simulink model "EST"  (R2024b)
settings: Solver=FixedStepAuto  StartTime=0.0  StopTime=stopt  FixedStep=deltat  MaxStep=0.05  RelTol=1e-3
InitFcn:
  | clear all;
  | close all;
  | clc;
  | 
  | % add the data and script directories
  | addpath('data','scripts');
  | 
  | % load the constants (units)
  | constants;
  | 
  | % load the simulation parameters
  | preprocessing;
StopFcn:
  | postprocessing;
values from neighbouring files (symbols this model uses):
  deltat = 15*unit("min")    [preprocessing.m]
undefined symbols (not defined in the file or in its folder): aElectricityDemand, aElectricToThermal, aExtraction, aInjection, alphaDemandTransport, aThermalToElectric, ccSurroundingsDemandTransport, ccSurroundingsStorage, ccSurroundingsSupplyTransport, dFluidDemandTransport, dFluidSupplyTransport, dStorageMaterial, eStorage, EStorageInitial, EStorageMax, EStorageMin, irPipeDemandTransport, irPipeSupplyTransport, l1PipeSupplyTransport, l2PipeSupplyTransport, lDemandTransport, lPipeDemandTransport, lStorage, rInjection, rplDemandTransport, rStorage, shcFluidDemandTransport, shcFluidSupplyTransport, shcStorageMaterial, tcInsDemandTransport, tcInsSupplyTransport, tcPipeDemandTransport, tcPipeSupplyTransport, tcStorage, tFluidSupplyTransport, tInsDemandTransport, tInsSupplyTransport, tMinStorage, tPipeDemandTransport, tPipeSupplyTransport, tStorage, tSurroundingsStorage, tSurroundingsSupplyTransport, vFluidDemandTransport, vFluidSupplyTransport
settings Model: Creator=joche  LastModifiedBy=nanda
settings DataIOCC: SaveFormat=Array  SaveOutput=off  ReturnWorkspaceOutputs=off
settings OptimizationCC: ReuseModelBlockBuffer=off
settings ModelReferenceCC: EnableRefExpFcnMdlSchedulingChecks=on
settings RTWCC: GPUComputeCapability=3.5

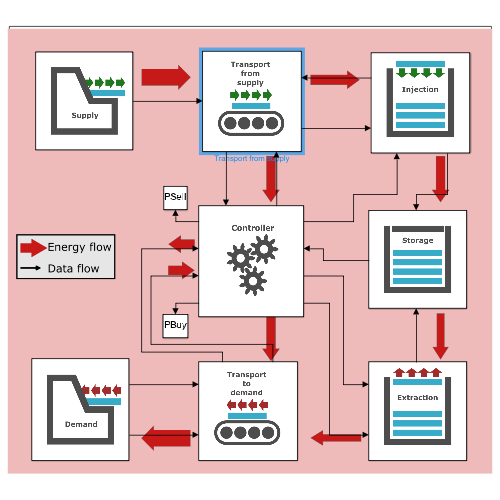
[thumbnail: Simulink's stored preview of the top-level diagram]
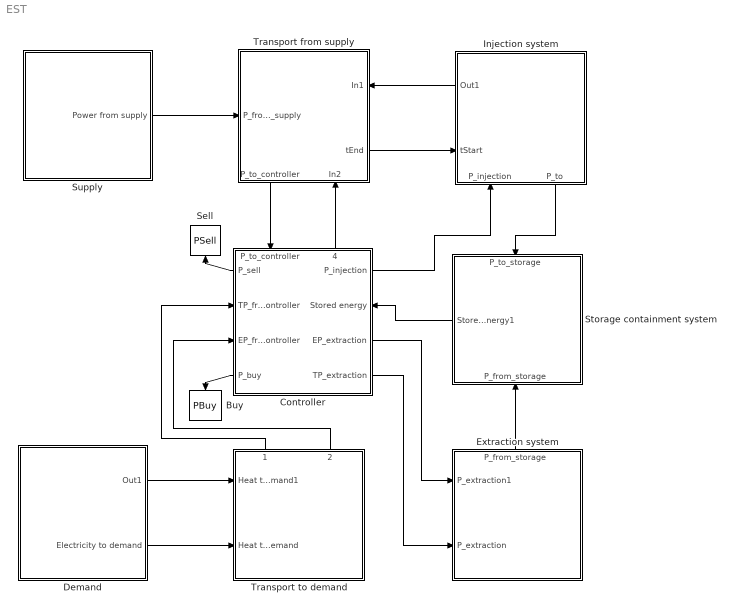
== system EST ==
  Buy : ToWorkspace  VariableName=PBuy  SampleTime=-1
  Controller : Subsystem
      settings: PortSchema="{\"entries\":[{\"content\":{\"sides\":[{\"content\":{\"connectorIds\":[\"Out5\",\"In1\",\"In2\",\"Out6\"]},\"type\":\"ConnectorPlacement.EquallySpacedRectSide\",\"uuid\":\"4656efb6-2d0d-4474-86b5-c32f145dee9d\"},{\"content\":{\"connectorIds\":[\"Out1\",\"In4\",\"Out2\",\"Out3\"],\"side\":\"RIGHT\"},\"type\":\"ConnectorPlacement.EquallySpacedRectSide\",\"uuid\":\"dff66aad-400a-439a-ac79-1f4b59d602b7\"},{\"content\":{\"connectorIds\":[\"In3\",\"Out4\"],\"side\":\"TOP\"},\"type\":\"ConnectorPlacement.EquallySpacedRectSide\",\"uuid\":\"e3dc4f2c-bed2-4e2c-ac62-d9db3cbbe72b\"}]},\"type\":\"ConnectorPlacement.EquallySpacedConnector\",\"uuid\":\"8904561c-f713-42e5-8c86-14541e4bd2e4\"}],\"packageUris\":[\"http://schema.mathworks.com/mf0/Connector/R2020b\"],\"version\":\"1.0\"}"
      mask Display: image('$imagefile'); % Use "Edit Image" on toolstrip to change.
  Demand : Subsystem
      mask Display: image('$imagefile'); % Use "Edit Image" on toolstrip to change.
  Extraction system : Subsystem
      settings: PortSchema="{\"entries\":[{\"content\":{\"sides\":[{\"content\":{},\"type\":\"ConnectorPlacement.EquallySpacedRectSide\",\"uuid\":\"05c5933d-55fc-4e06-853f-fc26d42905f9\"},{\"content\":{\"connectorIds\":[\"In1\",\"In2\"],\"side\":\"RIGHT\"},\"type\":\"ConnectorPlacement.EquallySpacedRectSide\",\"uuid\":\"327426c5-31d5-498b-a2bd-83e49353408c\"},{\"content\":{\"side\":\"TOP\"},\"type\":\"ConnectorPlacement.EquallySpacedRectSide\",\"uuid\":\"55306cf3-a3de-4385-a5ae-b8600ecdd5a2\"},{\"content\":{\"connectorIds\":[\"Out1\"],\"side\":\"BOTTOM\"},\"type\":\"ConnectorPlacement.EquallySpacedRectSide\",\"uuid\":\"08fcc9c3-40d3-4ac6-b914-dfeef6039ffb\"}]},\"type\":\"ConnectorPlacement.EquallySpacedConnector\",\"uuid\":\"cb35d5ba-e8c6-462c-b7b2-fe8356d4b0a1\"}],\"packageUris\":[\"http://schema.mathworks.com/mf0/Connector/R2020b\"],\"version\":\"1.0\"}"
      mask Display: image('$imagefile'); % Use "Edit Image" on toolstrip to change.
  Injection system : Subsystem
      settings: PortSchema="{\"entries\":[{\"content\":{\"sides\":[{\"content\":{},\"type\":\"ConnectorPlacement.EquallySpacedRectSide\",\"uuid\":\"05c5933d-55fc-4e06-853f-fc26d42905f9\"},{\"content\":{\"connectorIds\":[\"In2\",\"Out1\"],\"side\":\"RIGHT\"},\"type\":\"ConnectorPlacement.EquallySpacedRectSide\",\"uuid\":\"327426c5-31d5-498b-a2bd-83e49353408c\"},{\"content\":{\"connectorIds\":[\"Out2\",\"In1\"],\"side\":\"TOP\"},\"type\":\"ConnectorPlacement.EquallySpacedRectSide\",\"uuid\":\"55306cf3-a3de-4385-a5ae-b8600ecdd5a2\"},{\"content\":{\"side\":\"BOTTOM\"},\"type\":\"ConnectorPlacement.EquallySpacedRectSide\",\"uuid\":\"08fcc9c3-40d3-4ac6-b914-dfeef6039ffb\"}]},\"type\":\"ConnectorPlacement.EquallySpacedConnector\",\"uuid\":\"cb35d5ba-e8c6-462c-b7b2-fe8356d4b0a1\"}],\"packageUris\":[\"http://schema.mathworks.com/mf0/Connector/R2020b\"],\"version\":\"1.0\"}"
      mask Display: image('$imagefile'); % Use "Edit Image" on toolstrip to change.
  Sell : ToWorkspace  VariableName=PSell  SampleTime=-1
  Storage containment system : Subsystem
      settings: PortSchema="{\"entries\":[{\"content\":{\"sides\":[{\"content\":{\"connectorIds\":[\"Out1\"]},\"type\":\"ConnectorPlacement.EquallySpacedRectSide\",\"uuid\":\"0ba48424-33b9-4934-970f-64fe5d8b070e\"},{\"content\":{\"side\":\"RIGHT\"},\"type\":\"ConnectorPlacement.EquallySpacedRectSide\",\"uuid\":\"9cde340f-8f39-4499-9a12-5e1623737660\"},{\"content\":{\"connectorIds\":[\"In1\"],\"side\":\"TOP\"},\"type\":\"ConnectorPlacement.EquallySpacedRectSide\",\"uuid\":\"2af8db04-7fd0-4902-8637-8dc00edb4598\"},{\"content\":{\"connectorIds\":[\"In2\"],\"side\":\"BOTTOM\"},\"type\":\"ConnectorPlacement.EquallySpacedRectSide\",\"uuid\":\"e21ea806-d777-41a3-a53f-556fae66854b\"}]},\"type\":\"ConnectorPlacement.EquallySpacedConnector\",\"uuid\":\"4e2ddb36-4db3-4ab4-858b-ebb8ccefeb1f\"}],\"packageUris\":[\"http://schema.mathworks.com/mf0/Connector/R2020b\"],\"version\":\"1.0\"}"
      mask Display: image('$imagefile'); % Use "Edit Image" on toolstrip to change.
  Supply : Subsystem
      mask Display: image('$imagefile'); % Use "Edit Image" on toolstrip to change.
  Transport from supply : Subsystem
      settings: PortSchema="{\"entries\":[{\"content\":{\"sides\":[{\"content\":{\"connectorIds\":[\"In1\"]},\"type\":\"ConnectorPlacement.EquallySpacedRectSide\",\"uuid\":\"31329006-3d36-4d93-9c44-7503a515d397\"},{\"content\":{\"connectorIds\":[\"In3\",\"Out1\"],\"side\":\"RIGHT\"},\"type\":\"ConnectorPlacement.EquallySpacedRectSide\",\"uuid\":\"aba139c7-f9b6-4881-a56b-a4cbbedacd88\"},{\"content\":{\"side\":\"TOP\"},\"type\":\"ConnectorPlacement.EquallySpacedRectSide\",\"uuid\":\"e683eb73-7a35-4160-9c39-da83856a6278\"},{\"content\":{\"connectorIds\":[\"Out2\",\"In2\"],\"side\":\"BOTTOM\"},\"type\":\"ConnectorPlacement.EquallySpacedRectSide\",\"uuid\":\"1170dd18-447c-437f-9043-6812c2877331\"}]},\"type\":\"ConnectorPlacement.EquallySpacedConnector\",\"uuid\":\"804af608-1d70-444f-af69-e05f19bf98f3\"}],\"packageUris\":[\"http://schema.mathworks.com/mf0/Connector/R2020b\"],\"version\":\"1.0\"}"
      mask Display: image('$imagefile'); % Use "Edit Image" on toolstrip to change.
  Transport to demand : Subsystem
      settings: PortSchema="{\"entries\":[{\"content\":{\"sides\":[{\"content\":{\"connectorIds\":[\"In1\",\"In2\"]},\"type\":\"ConnectorPlacement.EquallySpacedRectSide\",\"uuid\":\"31329006-3d36-4d93-9c44-7503a515d397\"},{\"content\":{\"side\":\"RIGHT\"},\"type\":\"ConnectorPlacement.EquallySpacedRectSide\",\"uuid\":\"aba139c7-f9b6-4881-a56b-a4cbbedacd88\"},{\"content\":{\"connectorIds\":[\"Out1\",\"Out2\"],\"side\":\"TOP\"},\"type\":\"ConnectorPlacement.EquallySpacedRectSide\",\"uuid\":\"e683eb73-7a35-4160-9c39-da83856a6278\"},{\"content\":{\"side\":\"BOTTOM\"},\"type\":\"ConnectorPlacement.EquallySpacedRectSide\",\"uuid\":\"c378138f-7233-4483-870c-40a69b3495ee\"}]},\"type\":\"ConnectorPlacement.EquallySpacedConnector\",\"uuid\":\"804af608-1d70-444f-af69-e05f19bf98f3\"}],\"packageUris\":[\"http://schema.mathworks.com/mf0/Connector/R2020b\"],\"version\":\"1.0\"}"
      mask Display: image('$imagefile'); % Use "Edit Image" on toolstrip to change.
  wires:
  Supply/1(Power from supply) -> Transport from supply/1(P_from_supply)
  Transport from supply/2(P_to_controller) -> Controller/3(P_to_controller)
  Transport to demand/1(P_from_controler) -> Controller/1(TP_from_controller)
  Demand/1(Out1) -> Transport to demand/1(Heat to demand1)
  Controller/3(TP_extraction) -> Extraction system/1(P_extraction)
  Injection system/2(P_to) -> Storage containment system/1(P_to_storage)
  Extraction system/1(P_from_storage) -> Storage containment system/2(P_from_storage)
  Storage containment system/1(Stored energy1) -> Controller/4(Stored energy)
  Controller/1(P_injection) -> Injection system/1(P_injection)
  Controller/6(P_buy) -> Buy/1
  Transport from supply/1(tEnd) -> Injection system/2(tStart)
  Controller/5(P_sell) -> Sell/1
  Injection system/1(Out1) -> Transport from supply/3(In1)
  Demand/2(Electricity to demand) -> Transport to demand/2(Heat to demand)
  Transport to demand/2(P_from_controler1) -> Controller/2(EP_from_controller)
  Controller/2(EP_extraction) -> Extraction system/2(P_extraction1)
  Controller/4(TP_sold_from_pipes) -> Transport from supply/2(In2)

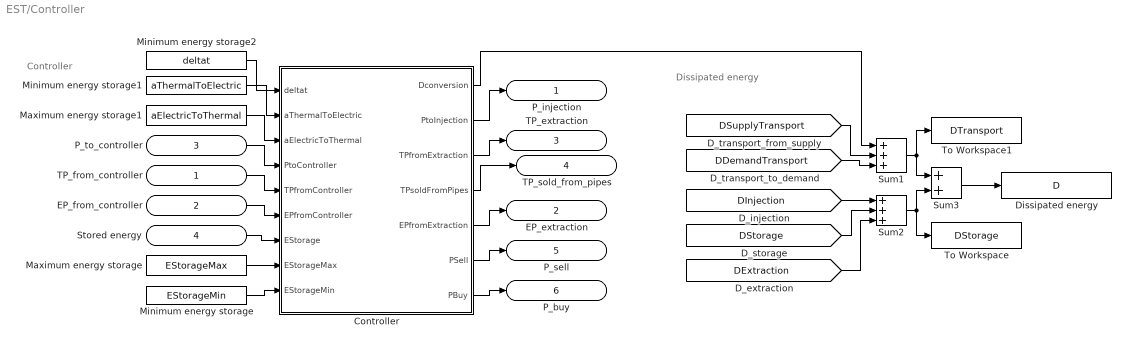
== system EST/Controller ==
  note: Dissipated energy
  note: Controller
  TP_from_controller : Inport
  EP_from_controller : Inport  Port=2
  P_to_controller : Inport  Port=3
  Stored energy : Inport  Port=4
  Controller : MATLAB Function  TreatAsAtomicUnit=on
  Dissipated energy : ToWorkspace  VariableName=D  SampleTime=-1
  Maximum energy storage : Constant  Value=EStorageMax
  Maximum energy storage1 : Constant  Value=aElectricToThermal
  Minimum energy storage : Constant  Value=EStorageMin
  Minimum energy storage1 : Constant  Value=aThermalToElectric
  Minimum energy storage2 : Constant  Value=deltat
  Sum1 : Sum  Inputs=+++
  Sum2 : Sum  Inputs=+++
  Sum3 : Sum
  To Workspace : ToWorkspace  VariableName=DStorage  SampleTime=-1
  To Workspace1 : ToWorkspace  VariableName=DTransport  SampleTime=-1
  P_injection : Outport
  EP_extraction : Outport  Port=2
  TP_extraction : Outport  Port=3
  TP_sold_from_pipes : Outport  Port=4
  P_sell : Outport  Port=5
  P_buy : Outport  Port=6
  wires:
  TP_from_controller/1 -> Controller/5(TPfromController)
  Controller/3(TPfromExtraction) -> TP_extraction/1
  Controller/6(PSell) -> P_sell/1
  Controller/7(PBuy) -> P_buy/1
  Minimum energy storage/1 -> Controller/9(EStorageMin)
  Maximum energy storage/1 -> Controller/8(EStorageMax)
  P_to_controller/1 -> Controller/4(PtoController)
  Controller/2(PtoInjection) -> P_injection/1
  Stored energy/1 -> Controller/7(EStorage)
  [DDemandTransport] -> Sum1/3
  [DSupplyTransport] -> Sum1/2
  [DInjection] -> Sum2/1
  [DStorage] -> Sum2/2
  [DExtraction] -> Sum2/3
  Sum2/1 -> To Workspace/1, Sum3/2
  Sum1/1 -> To Workspace1/1, Sum3/1
  Sum3/1 -> Dissipated energy/1
  EP_from_controller/1 -> Controller/6(EPfromController)
  Controller/5(EPfromExtraction) -> EP_extraction/1
  Maximum energy storage1/1 -> Controller/3(aElectricToThermal)
  Minimum energy storage1/1 -> Controller/2(aThermalToElectric)
  Controller/1(Dconversion) -> Sum1/1
  Minimum energy storage2/1 -> Controller/1(deltat)
  Controller/4(TPsoldFromPipes) -> TP_sold_from_pipes/1

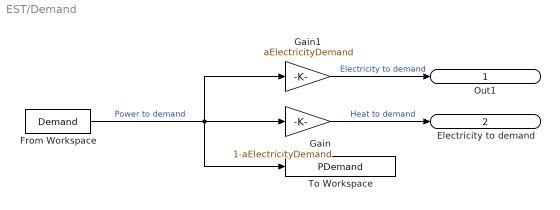
== system EST/Demand ==
  From Workspace : FromWorkspace  VariableName=Demand  OutputAfterFinalValue=Setting to zero
  Gain : Gain  Gain=1-aElectricityDemand
  Gain1 : Gain  Gain=aElectricityDemand
  To Workspace : ToWorkspace  VariableName=PDemand  SampleTime=-1
  Out1 : Outport
  Electricity to demand : Outport  Port=2
  wires:
  From Workspace/1 -> Gain/1, Gain1/1, To Workspace/1  "Power to demand"
  Gain/1 -> Electricity to demand/1  "Heat to demand"
  Gain1/1 -> Out1/1  "Electricity to demand"

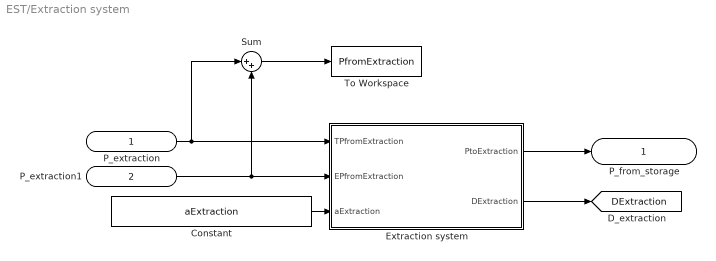
== system EST/Extraction system ==
  P_extraction : Inport
  P_extraction1 : Inport  Port=2
  Constant : Constant  Value=aExtraction
  Extraction system : MATLAB Function  TreatAsAtomicUnit=on
  Sum : Sum  Inputs=|++
  To Workspace : ToWorkspace  VariableName=PfromExtraction  SampleTime=-1
  P_from_storage : Outport
  tag scope: DExtraction=global
  wires:
  P_extraction/1 -> Sum/1, Extraction system/1(TPfromExtraction)
  Extraction system/1(PtoExtraction) -> P_from_storage/1
  Extraction system/2(DExtraction) -> [DExtraction]
  Constant/1 -> Extraction system/3(aExtraction)
  P_extraction1/1 -> Extraction system/2(EPfromExtraction), Sum/2
  Sum/1 -> To Workspace/1

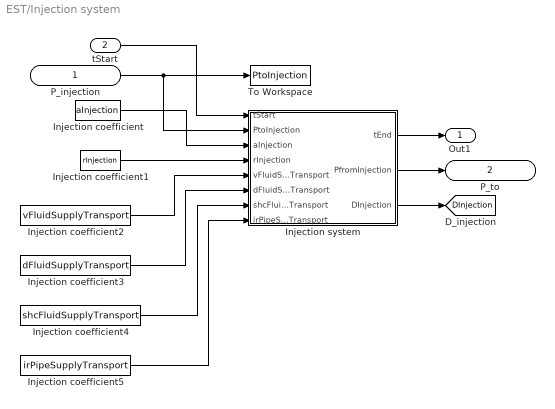
== system EST/Injection system ==
  P_injection : Inport
  tStart : Inport  Port=2
  Injection coefficient : Constant  Value=aInjection
  Injection coefficient1 : Constant  Value=rInjection
  Injection coefficient2 : Constant  Value=vFluidSupplyTransport
  Injection coefficient3 : Constant  Value=dFluidSupplyTransport
  Injection coefficient4 : Constant  Value=shcFluidSupplyTransport
  Injection coefficient5 : Constant  Value=irPipeSupplyTransport
  Injection system : MATLAB Function  TreatAsAtomicUnit=on
  To Workspace : ToWorkspace  VariableName=PtoInjection  SampleTime=-1
  Out1 : Outport
  P_to : Outport  Port=2
  tag scope: DInjection=global
  wires:
  Injection coefficient4/1 -> Injection system/7(shcFluidSupplyTransport)
  Injection coefficient1/1 -> Injection system/4(rInjection)
  tStart/1 -> Injection system/1(tStart)
  P_injection/1 -> To Workspace/1, Injection system/2(PtoInjection)
  Injection coefficient/1 -> Injection system/3(aInjection)
  Injection coefficient2/1 -> Injection system/5(vFluidSupplyTransport)
  Injection coefficient3/1 -> Injection system/6(dFluidSupplyTransport)
  Injection coefficient5/1 -> Injection system/8(irPipeSupplyTransport)
  Injection system/1(tEnd) -> Out1/1
  Injection system/2(PfromInjection) -> P_to/1
  Injection system/3(DInjection) -> [DInjection]

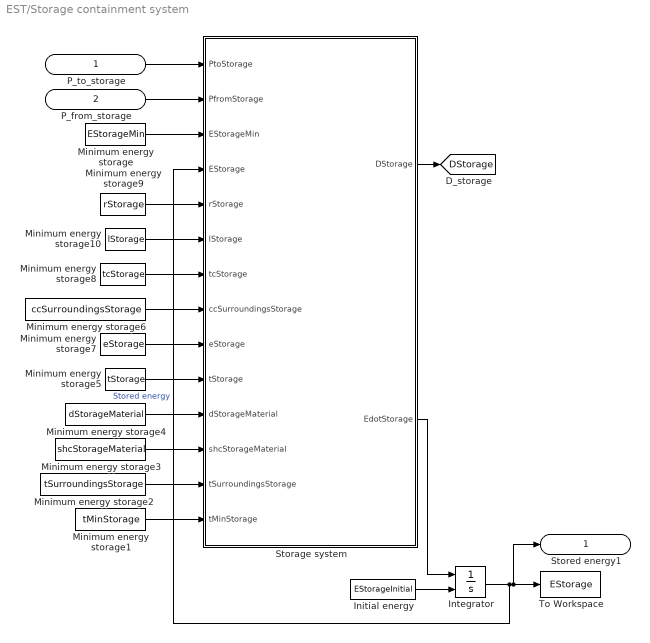
== system EST/Storage containment system ==
  P_to_storage : Inport
  P_from_storage : Inport  Port=2
  Initial energy : Constant  Value=EStorageInitial
  Integrator : Integrator  InitialConditionSource=external
  Minimum energy storage : Constant  Value=EStorageMin
  Minimum energy storage1 : Constant  Value=tMinStorage
  Minimum energy storage10 : Constant  Value=lStorage
  Minimum energy storage2 : Constant  Value=tSurroundingsStorage
  Minimum energy storage3 : Constant  Value=shcStorageMaterial
  Minimum energy storage4 : Constant  Value=dStorageMaterial
  Minimum energy storage5 : Constant  Value=tStorage
  Minimum energy storage6 : Constant  Value=ccSurroundingsStorage
  Minimum energy storage7 : Constant  Value=eStorage
  Minimum energy storage8 : Constant  Value=tcStorage
  Minimum energy storage9 : Constant  Value=rStorage
  Storage system : MATLAB Function  TreatAsAtomicUnit=on
  To Workspace : ToWorkspace  VariableName=EStorage  SampleTime=-1
  Stored energy1 : Outport
  tag scope: DStorage=global
  wires:
  P_from_storage/1 -> Storage system/2(PfromStorage)
  Initial energy/1 -> Integrator/2
  P_to_storage/1 -> Storage system/1(PtoStorage)
  Minimum energy storage3/1 -> Storage system/12(shcStorageMaterial)
  Minimum energy storage/1 -> Storage system/3(EStorageMin)
  Minimum energy storage7/1 -> Storage system/9(eStorage)
  Minimum energy storage2/1 -> Storage system/13(tSurroundingsStorage)
  Minimum energy storage6/1 -> Storage system/8(ccSurroundingsStorage)
  Minimum energy storage5/1 -> Storage system/10(tStorage)
  Minimum energy storage10/1 -> Storage system/6(lStorage)
  Minimum energy storage8/1 -> Storage system/7(tcStorage)
  Minimum energy storage9/1 -> Storage system/5(rStorage)
  Minimum energy storage1/1 -> Storage system/14(tMinStorage)
  Minimum energy storage4/1 -> Storage system/11(dStorageMaterial)
  Storage system/1(DStorage) -> [DStorage]
  Storage system/2(EdotStorage) -> Integrator/1
  Integrator/1 -> To Workspace/1, Stored energy1/1, Storage system/4(EStorage)  "Stored energy"

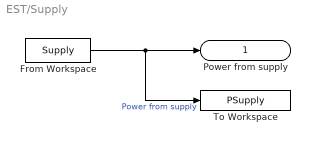
== system EST/Supply ==
  From Workspace : FromWorkspace  VariableName=Supply
  To Workspace : ToWorkspace  VariableName=PSupply  SampleTime=-1
  Power from supply : Outport
  wires:
  From Workspace/1 -> To Workspace/1, Power from supply/1  "Power from supply"

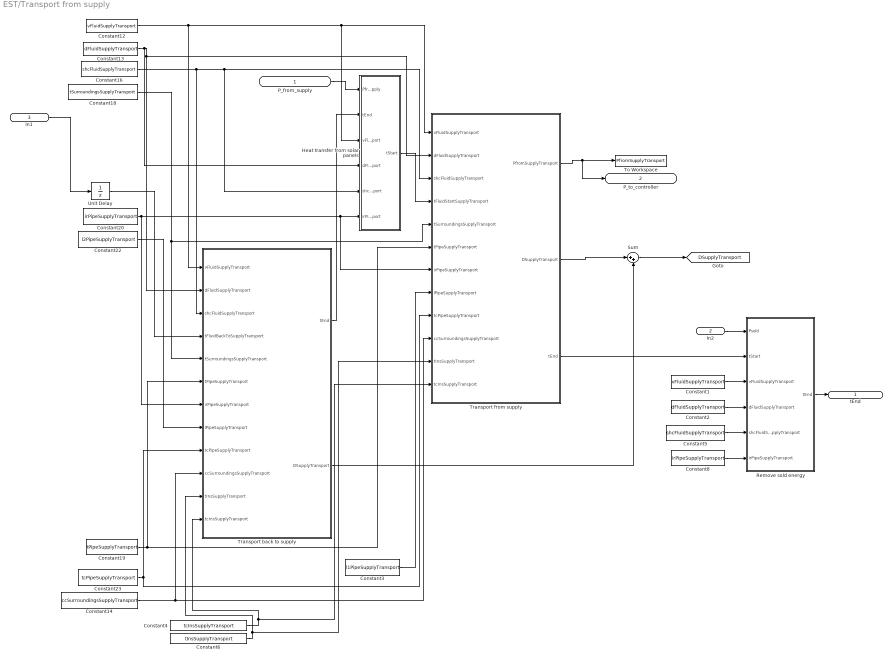
== system EST/Transport from supply ==
  P_from_supply : Inport
  In2 : Inport  Port=2
  In1 : Inport  Port=3
  Constant1 : Constant  Value=vFluidSupplyTransport
  Constant12 : Constant  Value=vFluidSupplyTransport
  Constant13 : Constant  Value=dFluidSupplyTransport
  Constant14 : Constant  Value=ccSurroundingsSupplyTransport
  Constant16 : Constant  Value=shcFluidSupplyTransport
  Constant18 : Constant  Value=tSurroundingsSupplyTransport
  Constant19 : Constant  Value=tPipeSupplyTransport
  Constant2 : Constant  Value=dFluidSupplyTransport
  Constant20 : Constant  Value=irPipeSupplyTransport
  Constant22 : Constant  Value=l2PipeSupplyTransport
  Constant23 : Constant  Value=tcPipeSupplyTransport
  Constant3 : Constant  Value=l1PipeSupplyTransport
  Constant4 : Constant  Value=tcInsSupplyTransport
  Constant5 : Constant  Value=shcFluidSupplyTransport
  Constant6 : Constant  Value=tInsSupplyTransport
  Constant8 : Constant  Value=irPipeSupplyTransport
  Heat transfer from solar panels : MATLAB Function  TreatAsAtomicUnit=on
  Remove sold energy : MATLAB Function  TreatAsAtomicUnit=on
  Sum : Sum  Inputs=|++
  To Workspace : ToWorkspace  VariableName=PfromSupplyTransport  SampleTime=-1
  Transport back to supply : MATLAB Function  TreatAsAtomicUnit=on
  Transport from supply : MATLAB Function  TreatAsAtomicUnit=on
  Unit Delay : UnitDelay  InitialCondition=tFluidSupplyTransport  SampleTime=-1  HasFrameUpgradeWarning=on
  tEnd : Outport
  P_to_controller : Outport  Port=2
  tag scope: DSupplyTransport=global
  wires:
  In1/1 -> Unit Delay/1
  Constant16/1 -> Heat transfer from solar panels/5(shcFluidSupplyTransport), Transport from supply/3(shcFluidSupplyTransport), Transport back to supply/3(shcFluidSupplyTransport)
  Constant22/1 -> Transport back to supply/8(lPipeSupplyTransport)
  Transport from supply/1(PfromSupplyTransport) -> To Workspace/1, P_to_controller/1
  P_from_supply/1 -> Heat transfer from solar panels/1(PfromSupply)
  Constant14/1 -> Transport from supply/10(ccSurroundingsSupplyTransport), Transport back to supply/10(ccSurroundingsSupplyTransport)
  Constant20/1 -> Transport from supply/7(irPipeSupplyTransport), Heat transfer from solar panels/6(irPipeSupplyTransport), Transport back to supply/7(irPipeSupplyTransport)
  Constant23/1 -> Transport from supply/9(tcPipeSupplyTransport), Transport back to supply/9(tcPipeSupplyTransport)
  Constant12/1 -> Heat transfer from solar panels/3(vFluidSupplyTransport), Transport from supply/1(vFluidSupplyTransport), Transport back to supply/1(vFluidSupplyTransport)
  Constant18/1 -> Transport from supply/5(tSurroundingsSupplyTransport), Transport back to supply/5(tSurroundingsSupplyTransport)
  Constant3/1 -> Transport from supply/8(lPipeSupplyTransport)
  Constant19/1 -> Transport from supply/6(tPipeSupplyTransport), Transport back to supply/6(tPipeSupplyTransport)
  Constant13/1 -> Transport from supply/2(dFluidSupplyTransport), Transport back to supply/2(dFluidSupplyTransport), Heat transfer from solar panels/4(dFluidSupplyTransport)
  Unit Delay/1 -> Transport back to supply/4(tFluidBackToSupplyTransport)
  Transport back to supply/1(tEnd) -> Heat transfer from solar panels/2(tEnd)
  Transport back to supply/2(DSupplyTransport) -> Sum/2
  Heat transfer from solar panels/1(tStart) -> Transport from supply/4(tFluidStartSupplyTransport)
  Transport from supply/2(DSupplyTransport) -> Sum/1
  Transport from supply/3(tEnd) -> Remove sold energy/2(tStart)
  In2/1 -> Remove sold energy/1(Psold)
  Constant1/1 -> Remove sold energy/3(vFluidSupplyTransport)
  Constant2/1 -> Remove sold energy/4(dFluidSupplyTransport)
  Constant5/1 -> Remove sold energy/5(shcFluidSupplyTransport)
  Constant8/1 -> Remove sold energy/6(irPipeSupplyTransport)
  Sum/1 -> [DSupplyTransport]
  Remove sold energy/1(tEnd) -> tEnd/1
  Constant4/1 -> Transport from supply/12(tcInsSupplyTransport), Transport back to supply/12(tcInsSupplyTransport)
  Constant6/1 -> Transport from supply/11(tInsSupplyTransport), Transport back to supply/11(tInsSupplyTransport)

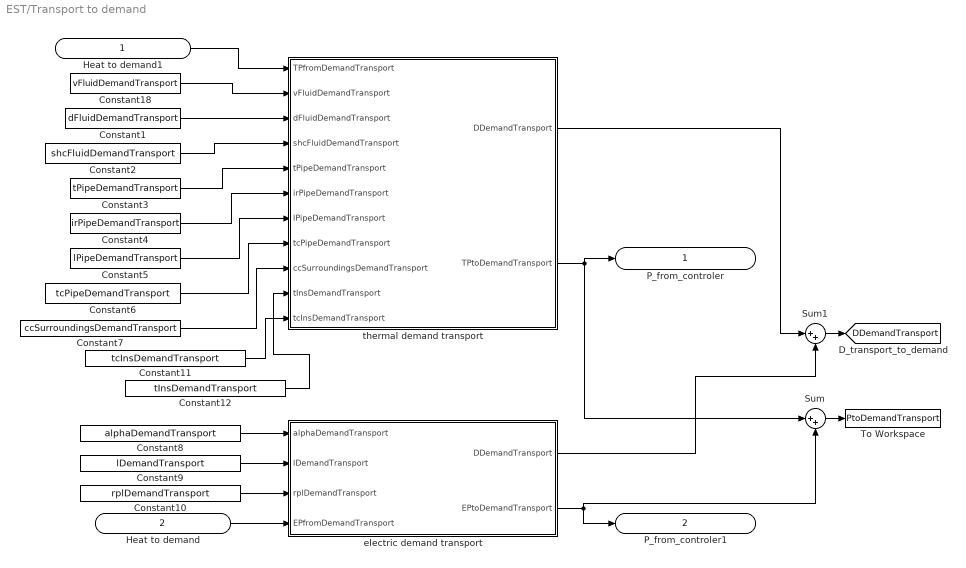
== system EST/Transport to demand ==
  Heat to demand1 : Inport
  Heat to demand : Inport  Port=2
  Constant1 : Constant  Value=dFluidDemandTransport
  Constant10 : Constant  Value=rplDemandTransport
  Constant11 : Constant  Value=tcInsDemandTransport
  Constant12 : Constant  Value=tInsDemandTransport
  Constant18 : Constant  Value=vFluidDemandTransport
  Constant2 : Constant  Value=shcFluidDemandTransport
  Constant3 : Constant  Value=tPipeDemandTransport
  Constant4 : Constant  Value=irPipeDemandTransport
  Constant5 : Constant  Value=lPipeDemandTransport
  Constant6 : Constant  Value=tcPipeDemandTransport
  Constant7 : Constant  Value=ccSurroundingsDemandTransport
  Constant8 : Constant  Value=alphaDemandTransport
  Constant9 : Constant  Value=lDemandTransport
  Sum : Sum  Inputs=|++
  Sum1 : Sum  Inputs=|++
  To Workspace : ToWorkspace  VariableName=PtoDemandTransport  SampleTime=-1
  electric demand transport : MATLAB Function  TreatAsAtomicUnit=on
  thermal demand transport : MATLAB Function  TreatAsAtomicUnit=on
  P_from_controler : Outport
  P_from_controler1 : Outport  Port=2
  tag scope: DDemandTransport=global
  wires:
  Heat to demand/1 -> electric demand transport/4(EPfromDemandTransport)
  Constant4/1 -> thermal demand transport/6(irPipeDemandTransport)
  Constant2/1 -> thermal demand transport/4(shcFluidDemandTransport)
  Constant18/1 -> thermal demand transport/2(vFluidDemandTransport)
  Constant6/1 -> thermal demand transport/8(tcPipeDemandTransport)
  Constant5/1 -> thermal demand transport/7(lPipeDemandTransport)
  Constant1/1 -> thermal demand transport/3(dFluidDemandTransport)
  Constant3/1 -> thermal demand transport/5(tPipeDemandTransport)
  Constant7/1 -> thermal demand transport/9(ccSurroundingsDemandTransport)
  thermal demand transport/1(DDemandTransport) -> Sum1/1
  thermal demand transport/2(TPtoDemandTransport) -> P_from_controler/1, Sum/1
  Heat to demand1/1 -> thermal demand transport/1(TPfromDemandTransport)
  Sum1/1 -> [DDemandTransport]
  electric demand transport/1(DDemandTransport) -> Sum1/2
  Sum/1 -> To Workspace/1
  electric demand transport/2(EPtoDemandTransport) -> Sum/2, P_from_controler1/1
  Constant8/1 -> electric demand transport/1(alphaDemandTransport)
  Constant9/1 -> electric demand transport/2(lDemandTransport)
  Constant10/1 -> electric demand transport/3(rplDemandTransport)
  Constant12/1 -> thermal demand transport/10(tInsDemandTransport)
  Constant11/1 -> thermal demand transport/11(tcInsDemandTransport)

== matlab function EST/Extraction system/Extraction system ==
  data: TPfromExtraction input; EPfromExtraction input; PtoExtraction output; DExtraction output; aExtraction input
function [PtoExtraction, DExtraction] = extraction(TPfromExtraction, EPfromExtraction, aExtraction)
    DExtraction = aExtraction / (1 - aExtraction) * EPfromExtraction;
    PtoExtraction = EPfromExtraction + DExtraction + TPfromExtraction;

== matlab function EST/Storage containment system/Storage system ==
  data: DStorage output; EdotStorage output; PtoStorage input; PfromStorage input; EStorageMin input; EStorage input; rStorage input; lStorage input; tcStorage input; ccSurroundingsStorage input; eStorage input; tStorage input; dStorageMaterial input; shcStorageMaterial input; tSurroundingsStorage input; tMinStorage input
function [DStorage, EdotStorage]= Storage(PtoStorage, PfromStorage, EStorageMin, EStorage,...
    rStorage, ...
    lStorage, ...
    tcStorage,...
    ccSurroundingsStorage, ...
    eStorage, ...
    tStorage, ...
    dStorageMaterial, ...
    shcStorageMaterial, ...
    tSurroundingsStorage,...
    tMinStorage) ...

    % Assume t << r, neglect radiation for now
    Atop = pi * rStorage .^ 2;
    Abottom = Atop;
    r0 = rStorage;
    r1 = r0 + tStorage;

    Rtop = rcondlinear(tcStorage, Atop, tStorage) ...
        + rconvlinear(ccSurroundingsStorage, Atop);

    Rbottom = rcondlinear(tcStorage, Abottom, tStorage) ...
        + rconvlinear(ccSurroundingsStorage, Abottom);
    
    Rside = rcondradial(r0, r1, tcStorage, lStorage) ...
        + rconvradial(ccSurroundingsStorage, lStorage, r1);

resistance = parallel(Rtop, Rbottom, Rside);
    
    vStorage = Atop * lStorage;

    dT = tMinStorage + (EStorage-EStorageMin) / (vStorage * dStorageMaterial * shcStorageMaterial) - tSurroundingsStorage;

    DStorage = dT / resistance;

    EdotStorage = PtoStorage - PfromStorage - DStorage;
end

function thermalResistance = rconvlinear(h, A)
    thermalResistance = 1 / (h*A);
end

function thermalResistance = rconvradial(h, L, R)
    thermalResistance = 1 / (2*pi*h*R*L);
end

function thermalResistance = rcondradial(ri, ro, k, L)
    thermalResistance = log(ro/ri)/(2*pi*k*L);
end

function thermalResistance = rcondlinear(k, A, L)
    thermalResistance = L/(k*A);
end

function thermalResistance = parallel(varargin)
    thermalResistance = 1 / sum(1 ./ [varargin{:}]);
end

function thermalResistance = rrad(e, A, T, Tenv)
    thermalResistance = 1 / (e * 5.67e-8 * A * (T.^2 + Tenv.^2) * (T + Tenv));
end

== matlab function EST/Transport from supply/Transport back to supply ==
  data: vFluidSupplyTransport input; dFluidSupplyTransport input; shcFluidSupplyTransport input; tFluidBackToSupplyTransport input; tSurroundingsSupplyTransport input; tPipeSupplyTransport input; irPipeSupplyTransport input; tEnd output; DSupplyTransport output; lPipeSupplyTransport input; tcPipeSupplyTransport input; ccSurroundingsSupplyTransport input; tInsSupplyTransport input; tcInsSupplyTransport input
function [tEnd, DSupplyTransport] = supplyTransport(vFluidSupplyTransport, ...
    dFluidSupplyTransport, ...
    shcFluidSupplyTransport, ...
    tFluidBackToSupplyTransport, ...
    tSurroundingsSupplyTransport, ...
    tPipeSupplyTransport, ...
    irPipeSupplyTransport, ...
    lPipeSupplyTransport, ...
    tcPipeSupplyTransport, ...
    ccSurroundingsSupplyTransport, ...
    tInsSupplyTransport, ...
    tcInsSupplyTransport)...

    r0 = irPipeSupplyTransport;
    r1 = r0 + tPipeSupplyTransport;
    r2 = r1 + tInsSupplyTransport;

    innerArea = pi * r0.^2;
    massFlow = vFluidSupplyTransport * dFluidSupplyTransport * innerArea;

    dT = tFluidBackToSupplyTransport - tSurroundingsSupplyTransport;

    thermalResistance = log(r1/r0)/(2 * pi * tcPipeSupplyTransport * lPipeSupplyTransport) ...
        + log(r2/r1)/(2 * pi * tcInsSupplyTransport * lPipeSupplyTransport) ...
        + 1/(2 * pi * ccSurroundingsSupplyTransport * r2 * lPipeSupplyTransport);

    tempLoss = dT * (1 - exp( -1/(massFlow*shcFluidSupplyTransport*thermalResistance) ));
    dissipation = massFlow * shcFluidSupplyTransport * tempLoss;

    DSupplyTransport = dissipation;
    tEnd = tFluidBackToSupplyTransport - tempLoss;
end

== matlab function EST/Transport to demand/electric demand transport ==
  data: alphaDemandTransport input; lDemandTransport input; rplDemandTransport input; EPfromDemandTransport input; DDemandTransport output; EPtoDemandTransport output
function [DDemandTransport, EPtoDemandTransport] = electricDemandTransport(alphaDemandTransport, lDemandTransport, rplDemandTransport, EPfromDemandTransport)
    pdDemandTransport = (1+alphaDemandTransport)*2*sqrt(lDemandTransport*rplDemandTransport*EPfromDemandTransport);

    a = lDemandTransport*rplDemandTransport/(pdDemandTransport^2);
    b = (2*lDemandTransport*rplDemandTransport*EPfromDemandTransport/(pdDemandTransport^2)-1);
    c = (lDemandTransport*rplDemandTransport*EPfromDemandTransport^2)/(pdDemandTransport^2);

    coefficients = [a b c];
    dissipations = roots(coefficients);
    dissipations = real(dissipations(dissipations > 0));
    DDemandTransport = min(dissipations);

    EPtoDemandTransport = EPfromDemandTransport + DDemandTransport;

== matlab function EST/Transport from supply/Heat transfer from solar panels ==
  data: PfromSupply input; tEnd input; tStart output; vFluidSupplyTransport input; dFluidSupplyTransport input; shcFluidSupplyTransport input; irPipeSupplyTransport input
function tStart = solarPanels(PfromSupply, ...
    tEnd,...
    vFluidSupplyTransport, ...
    dFluidSupplyTransport, ...
    shcFluidSupplyTransport, ...
    irPipeSupplyTransport)

    r0 = irPipeSupplyTransport;
    innerArea = pi * r0.^2;
    massFlow = vFluidSupplyTransport * dFluidSupplyTransport * innerArea;

    
    tStart = tEnd+(PfromSupply)/(massFlow*shcFluidSupplyTransport);

== matlab function EST/Transport from supply/Remove sold energy ==
  data: Psold input; tStart input; tEnd output; vFluidSupplyTransport input; dFluidSupplyTransport input; shcFluidSupplyTransport input; irPipeSupplyTransport input
function tEnd = removeSoldEnergy(Psold, ...
    tStart,...
    vFluidSupplyTransport, ...
    dFluidSupplyTransport, ...
    shcFluidSupplyTransport, ...
    irPipeSupplyTransport)

    r0 = irPipeSupplyTransport;
    innerArea = pi * r0.^2;
    massFlow = vFluidSupplyTransport * dFluidSupplyTransport * innerArea;

    tEnd = tStart - (Psold)/(massFlow*shcFluidSupplyTransport);

== matlab function EST/Transport to demand/thermal demand transport ==
  data: TPfromDemandTransport input; vFluidDemandTransport input; dFluidDemandTransport input; shcFluidDemandTransport input; tPipeDemandTransport input; irPipeDemandTransport input; lPipeDemandTransport input; tcPipeDemandTransport input; ccSurroundingsDemandTransport input; DDemandTransport output; TPtoDemandTransport output; tInsDemandTransport input; tcInsDemandTransport input
function [DDemandTransport, TPtoDemandTransport] = thermalDemandTransport(TPfromDemandTransport,...
    vFluidDemandTransport, ...
    dFluidDemandTransport, ...
    shcFluidDemandTransport, ...
    tPipeDemandTransport, ...
    irPipeDemandTransport, ...
    lPipeDemandTransport, ...
    tcPipeDemandTransport, ...
    ccSurroundingsDemandTransport, ...
    tInsDemandTransport, ...
    tcInsDemandTransport)...

    r0 = irPipeDemandTransport;
    r1 = r0 + tPipeDemandTransport;
    r2 = r1 + tInsDemandTransport;

    innerArea = pi * r0.^2;
    massFlow = vFluidDemandTransport * dFluidDemandTransport * innerArea;

    thermalResistance = log(r1/r0)/(2 * pi * tcPipeDemandTransport * lPipeDemandTransport) ...
        + log(r2/r1)/(2 * pi * tcInsDemandTransport * lPipeDemandTransport) ...
        + 1/(2 * pi * ccSurroundingsDemandTransport * r2 * lPipeDemandTransport);

    dT = TPfromDemandTransport / (massFlow * shcFluidDemandTransport * exp( -1/(massFlow*shcFluidDemandTransport*thermalResistance) ));
    tempLoss = dT * (1 - exp( -1/(massFlow*shcFluidDemandTransport*thermalResistance) ));
    
    DDemandTransport = massFlow * shcFluidDemandTransport * tempLoss;
    TPtoDemandTransport = DDemandTransport + TPfromDemandTransport;
end

== matlab function EST/Injection system/Injection system ==
  data: tStart input; tEnd output; PtoInjection input; PfromInjection output; DInjection output; aInjection input; rInjection input; vFluidSupplyTransport input; dFluidSupplyTransport input; shcFluidSupplyTransport input; irPipeSupplyTransport input
function [tEnd, PfromInjection, DInjection] = injection(tStart, ...
    PtoInjection, ...
    aInjection, ...
    rInjection,...
    vFluidSupplyTransport, ...
    dFluidSupplyTransport, ...
    shcFluidSupplyTransport, ...
    irPipeSupplyTransport)

    r0 = irPipeSupplyTransport;
    innerArea = pi * r0 ^ 2;
    massFlow = vFluidSupplyTransport * dFluidSupplyTransport * innerArea;

    DInjection = aInjection * PtoInjection;
    PbackToSupply = rInjection * PtoInjection;
    tEnd = tStart - (1 - rInjection - aInjection) * PtoInjection/(massFlow*shcFluidSupplyTransport);
    PfromInjection = PtoInjection - DInjection - PbackToSupply;

== matlab function EST/Transport from supply/Transport from supply ==
  data: PfromSupplyTransport output; vFluidSupplyTransport input; DSupplyTransport output; dFluidSupplyTransport input; shcFluidSupplyTransport input; tFluidStartSupplyTransport input; tSurroundingsSupplyTransport input; tPipeSupplyTransport input; irPipeSupplyTransport input; lPipeSupplyTransport input; tcPipeSupplyTransport input; ccSurroundingsSupplyTransport input; tEnd output; tInsSupplyTransport input; tcInsSupplyTransport input
function [PfromSupplyTransport, DSupplyTransport, tEnd] = supplyTransport(vFluidSupplyTransport, ...
    dFluidSupplyTransport, ...
    shcFluidSupplyTransport, ...
    tFluidStartSupplyTransport, ...
    tSurroundingsSupplyTransport, ...
    tPipeSupplyTransport, ...
    irPipeSupplyTransport, ...
    lPipeSupplyTransport, ...
    tcPipeSupplyTransport, ...
    ccSurroundingsSupplyTransport, ...
    tInsSupplyTransport, ...
    tcInsSupplyTransport)...

    r0 = irPipeSupplyTransport;
    r1 = r0 + tPipeSupplyTransport;
    r2 = r1 + tInsSupplyTransport;

    innerArea = pi * r0.^2;
    massFlow = vFluidSupplyTransport * dFluidSupplyTransport * innerArea;

    dT = tFluidStartSupplyTransport - tSurroundingsSupplyTransport;

    PinSupplyTransport = dT * shcFluidSupplyTransport * massFlow;

    thermalResistance = log(r1/r0)/(2 * pi * tcPipeSupplyTransport * lPipeSupplyTransport) ...
        + log(r2/r1)/(2 * pi * tcInsSupplyTransport * lPipeSupplyTransport) ...
        + 1/(2 * pi * ccSurroundingsSupplyTransport * r2 * lPipeSupplyTransport);

    tempLoss = dT * (1 - exp( -1/(massFlow*shcFluidSupplyTransport*thermalResistance) ));
    dissipation = massFlow * shcFluidSupplyTransport * tempLoss;

    DSupplyTransport = dissipation;
    PfromSupplyTransport = PinSupplyTransport - DSupplyTransport;
    tEnd = tFluidStartSupplyTransport - tempLoss;
end

== matlab function EST/Controller/Controller ==
  data: deltat input; Dconversion output; aThermalToElectric input; aElectricToThermal input; PtoInjection output; TPfromExtraction output; TPsoldFromPipes output; EPfromExtraction output; PSell output; PBuy output; PtoController input; TPfromController input; EPfromController input; EStorage input; EStorageMax input; EStorageMin input
function [Dconversion, PtoInjection, TPfromExtraction, TPsoldFromPipes, EPfromExtraction, PSell, PBuy] = controller(deltat, aThermalToElectric, aElectricToThermal, PtoController, TPfromController, EPfromController, EStorage, EStorageMax, EStorageMin)
    %% Power surplus or deficit
    EPtoController = 0;              % Electric energy that can be taken from the supply
    TPtoController = PtoController;  % Thermal energy that can be taken from the supply

    deltaTP = TPtoController - TPfromController;
    deltaEP = EPtoController - EPfromController;

    TPsoldFromPipes = 0.0;
    ERemainingInStorage = EStorage;
    %% Thermal excess
    if deltaTP >= 0
        % Convert thermal to electric
        EPconverted = min(deltaTP * (1 - aThermalToElectric), -deltaEP); % this much electricity can be substituted with thermal power
        EPtoController = EPtoController + EPconverted;
        deltaTP = deltaTP - EPconverted / (1 - aThermalToElectric);
        Dconversion = EPconverted / (1 - aThermalToElectric) * aThermalToElectric;

        % store thermal needed
        if EStorage < EStorageMax 
            PtoInjection = min(deltaTP, (EStorageMax - EStorage)/deltat);
        else
            PtoInjection = 0;
        end

        % sell rest of thermal
        TPsoldFromPipes = deltaTP - PtoInjection;
        PSell = aThermalToElectric * TPsoldFromPipes;
        PBuy = 0;
        TPfromExtraction = 0;
    %% Thermal deficit
    else
        %% Storage injection

        PtoInjection = 0;

        %% Storage extraction

        % Storage system is not empty
        if ERemainingInStorage > EStorageMin
            TPfromExtraction = min(-deltaTP, (ERemainingInStorage - EStorageMin)/deltat);
            ERemainingInStorage = ERemainingInStorage - TPfromExtraction*deltat;
        else
            TPfromExtraction = 0;
        end

        %% Load-balancing

        PSell = 0;
        ThermalDeficit = (-deltaTP - TPfromExtraction);
        ThermalDeficitInElectricity = ThermalDeficit / (1 - aElectricToThermal);
        Dconversion = ThermalDeficitInElectricity * aElectricToThermal;
        PBuy = ThermalDeficitInElectricity;
    end

    %% Handle electric deficit
    deltaEP = EPtoController - EPfromController;

    %% Storage extraction
    % Storage system is not empty
    if ERemainingInStorage > EStorageMin

        EPfromExtraction = min(max(-deltaEP,0), (ERemainingInStorage - EStorageMin)/deltat);
        ERemainingInStorage = ERemainingInStorage - EPfromExtraction*deltat;
    else

        EPfromExtraction = 0;

    end

    %% Load-balancing

    PSell = PSell + 0;
    EPremainingDeficit = max(0, -deltaEP - EPfromExtraction);
    PBuy = PBuy + EPremainingDeficit;
